simulink library "Lib_Turbo_TurbineNPSS_TMATS_org"  (Simulink 10.0)
settings: Solver=ode45  StartTime=0.0  StopTime=10.0  RelTol=1e-3  EnableMultiTasking=on
undefined symbols (not defined in the file): stripchar_TMATS
libraries: Lib_Solve_DataOut_TMATS x1
Description:
  | Thomas Modules
settings Model: Creator=jwchapm2  LastModifiedBy=annonymous

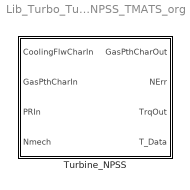
== system Lib_Turbo_TurbineNPSS_TMATS_org ==
  Turbine_NPSS : Subsystem  mask(T-MATS: Turbine, NPSS Library Block){X_T_Map_PRVec_M=[ 3.000  8.000], Y_T_Map_NcVec_M=[60 80  110], T_T_Map_WcArray_M=[0 0;0 0; 0 0], T_T_Map_EffArray_M=[0 0; 0 0; 0 0], s_T_Nc_M=0.0243, s_T_Wc_M=0.4504, s_T_PR_M=0.9736, s_T_Eff_M=0.9984, ConfigNPSS_M=1, Scale_M=none, CFlwEn_M=off, T_CoolFlwPos_M=0, iDesign_M=2, NcDes_M=100, EffDes_M=0.9328, PRDes_M=5, NDes_M=10000, FVar_M=strcat('iDes_',stripchar_TMATS(gcb),'.bin'), BlkNm_M=double(gcb), HP_M=off}
      mask prompts: X_T_Map_PRVec_M "X_T_Map_PRVec_M - Turbine Map Pressure Ratio Vector (X-axis)(nx1)"; Y_T_Map_NcVec_M "Y_T_Map_NcVec_M - Turbine Map Corrected Speed Vector (Y-axis)(mx1)"; T_T_Map_WcArray_M "T_T_Map_WcArray_M - Turbine Map Flow Array (Wc=f(Nc,PR))(mxn)"; T_T_Map_EffArray_M "T_T_Map_EffArray_M - Turbine Map Efficiency Array (Eff = f(Nc,PR))(mxn)"; s_T_Nc_M "s_T_Nc_M - Corrected Speed Scalar Constant (T_Nc)"; s_T_Wc_M "s_T_Wc_M - Flow Scalar Constant (T_Wc)"; s_T_PR_M "s_T_PR_M - Pressure Ratio Scalar Constant (T_PR)"; s_T_Eff_M "s_T_Eff_M - Efficiency Scalar Constant (T_Eff)"; ConfigNPSS_M "ConfigNPSS_M - configure for type usage of maps and constants"; Scale_M "Scalars"; CFlwEn_M "CFlwEn_M - Cooling Flow Enable [0-off, 1-on]"; T_CoolFlwPos_M "T_CoolFlwPos_M - Cooling Flow position [0 at inlet,  1 at exit] (cx1)"; iDesign_M "iDesign_M - Design fork (0 - Enable iDes, 1 - Use iDes Scalars, 2 - Use Specified Input Scalars)"; NcDes_M "NcDes_M - map Design Corrected Shaft Speed [rpm]"; EffDes_M "EffDes_M - Design Efficiency [frac]"; PRDes_M "PRDes_M - map Design Pressure Ratio [frac]"; NDes_M "NDes_M - Design Shaft Speed [rpm]"; FVar_M "FVar_M - File name for iDes Variables"; BlkNm_M "Block name as double for Simulink output"; HP_M "HP_M - Enable Health Parameter input (2x1 vector)"
      mask help: This block simulates the performance of a turbine using basic thermodynamic equations, properties, and table lookups. This block has been updated to be more similar to the baseline NPSS turbine module. Updates include removing the standard day components of the Nc and Wc calculations and updating the Flow error term to use input flow only, which translates to a turbine map in which Wc is defined as input flow only.
      mask init:
      | if iDesign_M == 1
      |     P = load(FVar_M);
      |     s_T_Nc_M = P(1);
      |     s_T_Wc_M = P(2);
      |     s_T_PR_M = P(3);
      |     s_T_Eff_M = P(4);
      | end
      | 
      | if length(X_T_Map_PRVec_M) ~= size(T_T_Map_WcArray_M,2)
      |     warning('number of columns in T_T_Map_WcArray_M does not match length of X_T_Map_PRVec_M');
      | end
      | if length(X_T_Map_PRVec_M) ~= size(T_T_Map_EffArray_M,2)
      |     warning('number of columns in T_T_Map_EffArray_M does not match length of X_T_Map_PRVec_M');
      | end
      | if length(Y_T_Map_NcVec_M) ~= size(T_T_Map_WcArray_M,1)
      |     warning('number of rows in T_T_Map_WcArray_M does not match length of Y_T_Map_NcVec_M');
      | end
      | if length(Y_T_Map_NcVec_M) ~= size(T_T_Map_EffArray_M,1)
      |     warning('number of rows in T_T_Map_EffArray_M does not match length of Y_T_Map_NcVec_M');
      | end
      | 
      | % produce warning if Health Parameters are enabled and IDesign is set to 0
      | if HP_M && iDesign_M == 0
      |     warning('iDesign is set to 0 (model on design) and health parameters are enabled. HP values will be ignored.');
      | end
      | 
      | %Manage Health Parameter inputs
      | if HP_M == 1
      |     if strcmp(get_param([BlkNm_M '/HP_Mods'],'BlockType'),'Constant')
      |         MSK_ReplaceBlock_TMATS([BlkNm_M '/HP_Mods'],'built-in/Inport');
      |     end
      |     set_param([BlkNm_M '/HP_Mods'],'Port',num2str(5));
      | elseif HP_M == 0
      |     if strcmp(get_param([BlkNm_M '/HP_Mods'],'BlockType'),'Inport')
      |         MSK_ReplaceBlock_TMATS([BlkNm_M '/HP_Mods'],'built-in/Constant');
      |         set_param([BlkNm_M '/HP_Mods'],'Value','[0, 0]');
      |     end
      | end
      mask Help: web(which('Turbo_TMATS_TrbNPSS.html'),'-helpbrowser')
      mask TypeOptions Scale_M: none | user defined | iDesign
      mask Callback CFlwEn_M: MSK_SEC_Enables_TMATS('CFlwEn_M',12,'en')
      mask Callback iDesign_M:
      | MSK_SEC_Enables_Ides_TMATS('iDesign_M',[5 6 7 8],'G1')
      | MSK_SEC_Enables_Ides_TMATS('iDesign_M',[14 15 16 17],'G2')
      | MSK_SEC_Enables_Ides_TMATS('iDesign_M',[18],'G3')
      mask DialogControl Control2 Prompt: Plot Map
      mask DialogControl Control2 Callback: MSK_PlotTMap_TMATS()

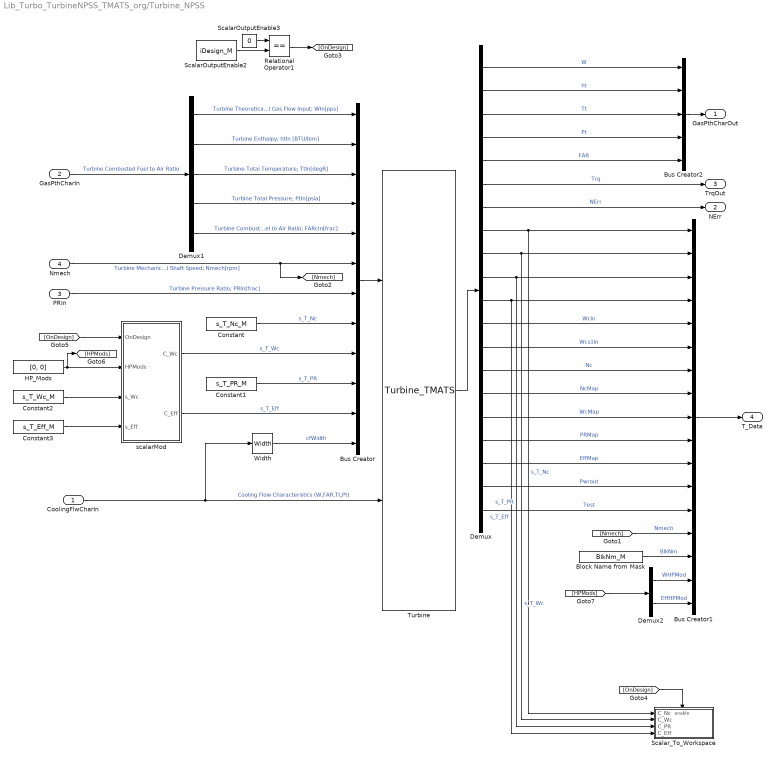
== system Lib_Turbo_TurbineNPSS_TMATS_org/Turbine_NPSS ==
  CoolingFlwCharIn : Inport
  GasPthCharIn : Inport  Port=2
  PRIn : Inport  Port=3
  Nmech : Inport  Port=4
  Block Name from Mask : Constant  Value=BlkNm_M
  Bus Creator : BusCreator  Inputs=12
  Bus Creator1 : BusCreator  Inputs=17
  Bus Creator2 : BusCreator  Inputs=5
  Constant : Constant  Value=s_T_Nc_M
  Constant1 : Constant  Value=s_T_PR_M
  Constant2 : Constant  Value=s_T_Wc_M
  Constant3 : Constant  Value=s_T_Eff_M
  Demux : Demux  Outputs=20
  Demux1 : Demux  Outputs=5
  Demux2 : Demux  Outputs=2
  HP_Mods : Constant  Value=[0, 0]
  Relational Operator1 : RelationalOperator  Operator===  OutDataTypeStr=boolean  RndMeth=Nearest
  ScalarOutputEnable2 : Constant  Value=iDesign_M
  ScalarOutputEnable3 : Constant  Value=0
  Scalar_To_Workspace : Subsystem
  Turbine : S-Function  FunctionName=Turbine_TMATS  Parameters=Y_T_Map_NcVec_M, X_T_Map_PRVec_M, T_T_Map_WcArray_M, T_T_Map_EffArray_M, T_CoolFlwPos_M, length(T_CoolFlwPos_M), CFlwEn_M, iDesign_M, NcDes_M, EffDes_M, PRDes_M, NDes_M, gcs, size(T_T_Map_WcArray_M,2), size(T_T_Map_EffArray_M,2), size(T_T_Map_WcArray_M,1), size(T_T_Map_EffArray_M,1), ConfigNPSS_M  SFunctionModules='h2tc_TMATS pt2sc_TMATS sp2tc_TMATS t2hc_TMATS interp2Ac_TMATS functions_TMATS'  SFunctionDeploymentMode=off  EnableBusSupport=off
  Width : Width
  scalarMod : Subsystem
  GasPthCharOut : Outport
  NErr : Outport  Port=2
  TrqOut : Outport  Port=3
  T_Data : Outport  Port=4
  wires:
  Demux/19 -> Bus Creator1/12  "Pwrout"
  Demux/18 -> Bus Creator1/11  "EffMap"
  Demux/17 -> Bus Creator1/10  "PRMap"
  Demux/16 -> Bus Creator1/9  "WcMap"
  Demux/15 -> Bus Creator1/8  "NcMap"
  Demux/14 -> Bus Creator1/7  "Nc"
  Demux/13 -> Bus Creator1/6  "Wcs1in"
  Demux/20 -> Bus Creator1/13  "Test"
  Width/1 -> Bus Creator/12  "cfWidth"
  Demux/11 -> Bus Creator1/4, Scalar_To_Workspace/4(C_Eff)  "s_T_Eff"
  Demux/10 -> Bus Creator1/3, Scalar_To_Workspace/3(C_PR)  "s_T_PR"
  Demux/9 -> Bus Creator1/2, Scalar_To_Workspace/2(C_Wc)  "s_T_Wc"
  Demux/8 -> Bus Creator1/1, Scalar_To_Workspace/1(C_Nc)  "s_T_Nc"
  Bus Creator1/1 -> T_Data/1
  Demux1/5 -> Bus Creator/5  "Turbine Combusted Fuel to Air Ratio; FARcIn[frac]"
  CoolingFlwCharIn/1 -> Turbine/2, Width/1  "Cooling Flow Characteristics (W,FAR,Tt,Pt)"
  Demux/7 -> NErr/1  "NErr"
  Demux1/1 -> Bus Creator/1  "Turbine Theoretical Gas Flow Input; WIn[pps]"
  GasPthCharIn/1 -> Demux1/1  "Turbine Combusted Fuel to Air Ratio"
  Bus Creator2/1 -> GasPthCharOut/1
  Demux1/4 -> Bus Creator/4  "Turbine Total Pressure; PtIn[psia]"
  Nmech/1 -> [Nmech], Bus Creator/6  "Turbine Mechanical Shaft Speed; Nmech[rpm]"
  Demux/6 -> TrqOut/1  "Trq"
  Demux/2 -> Bus Creator2/2  "ht"
  Bus Creator/1 -> Turbine/1
  Demux/4 -> Bus Creator2/4  "Pt"
  Demux/3 -> Bus Creator2/3  "Tt"
  Demux/5 -> Bus Creator2/5  "FAR"
  Demux/1 -> Bus Creator2/1  "W"
  Turbine/1 -> Demux/1
  Demux1/3 -> Bus Creator/3  "Turbine Total Temperature; TtIn[degR]"
  Demux1/2 -> Bus Creator/2  "Turbine Enthalpy; htIn [BTU/lbm]"
  PRIn/1 -> Bus Creator/7  "Turbine Pressure Ratio; PRIn[frac]"
  Demux/12 -> Bus Creator1/5  "Wcin"
  Block Name from Mask/1 -> Bus Creator1/15  "BlkNm"
  [Nmech] -> Bus Creator1/14  "Nmech"
  Constant/1 -> Bus Creator/8  "s_T_Nc"
  Constant1/1 -> Bus Creator/10  "s_T_PR"
  scalarMod/1(C_Wc) -> Bus Creator/9  "s_T_Wc"
  scalarMod/2(C_Eff) -> Bus Creator/11  "s_T_Eff"
  ScalarOutputEnable2/1 -> Relational Operator1/2
  ScalarOutputEnable3/1 -> Relational Operator1/1
  Relational Operator1/1 -> [OnDesign]
  [OnDesign] -> Scalar_To_Workspace/Enable
  HP_Mods/1 -> [HPMods], scalarMod/2(HPMods)
  [OnDesign] -> scalarMod/1(OnDesign)
  Constant2/1 -> scalarMod/3(s_Wc)
  Constant3/1 -> scalarMod/4(s_Eff)
  Demux2/1 -> Bus Creator1/16  "WHPMod"
  Demux2/2 -> Bus Creator1/17  "EffHPMod"
  [HPMods] -> Demux2/1

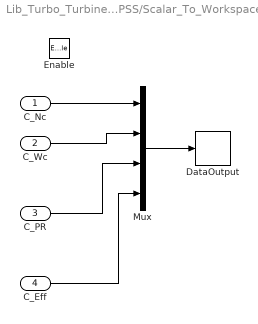
== system Lib_Turbo_TurbineNPSS_TMATS_org/Turbine_NPSS/Scalar_To_Workspace ==
  C_Nc : Inport
  C_Wc : Inport  Port=2
  C_PR : Inport  Port=3
  C_Eff : Inport  Port=4
  Enable : EnablePort
  DataOutput : Lib_Solve_DataOut_TMATS/DataOutput  FVar_M=double(FVar_M)
  Mux : Mux
  wires:
  Mux/1 -> DataOutput/1
  C_Eff/1 -> Mux/4
  C_PR/1 -> Mux/3
  C_Nc/1 -> Mux/1
  C_Wc/1 -> Mux/2

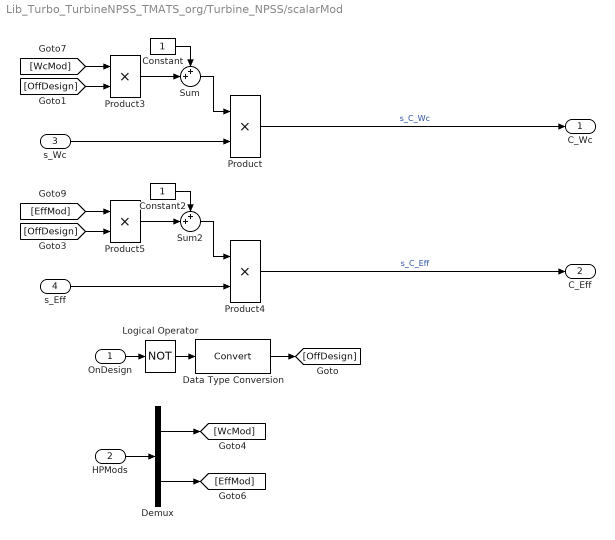
== system Lib_Turbo_TurbineNPSS_TMATS_org/Turbine_NPSS/scalarMod ==
  OnDesign : Inport
  HPMods : Inport  Port=2
  s_Wc : Inport  Port=3
  s_Eff : Inport  Port=4
  Constant : Constant
  Constant2 : Constant
  Data Type Conversion : DataTypeConversion
  Demux : Demux  Outputs=2
  Logical Operator : Logic  Operator=NOT  AllPortsSameDT=off  OutDataTypeStr=boolean
  Product{,3..5} (4 alike) : Product
  Sum : Sum  Inputs=++|
  Sum2 : Sum  Inputs=++|
  C_Wc : Outport
  C_Eff : Outport  Port=2
  wires:
  Demux/2 -> [EffMod]
  Demux/1 -> [WcMod]
  HPMods/1 -> Demux/1
  [OffDesign] -> Product5/2
  Product5/1 -> Sum2/2
  Constant2/1 -> Sum2/1
  [EffMod] -> Product5/1
  Sum2/1 -> Product4/1
  s_Eff/1 -> Product4/2
  [OffDesign] -> Product3/2
  Product3/1 -> Sum/2
  Constant/1 -> Sum/1
  [WcMod] -> Product3/1
  Sum/1 -> Product/1
  Logical Operator/1 -> Data Type Conversion/1
  Data Type Conversion/1 -> [OffDesign]
  OnDesign/1 -> Logical Operator/1
  s_Wc/1 -> Product/2
  Product/1 -> C_Wc/1  "s_C_Wc"
  Product4/1 -> C_Eff/1  "s_C_Eff"
